simulink model "Automotive_Performance_Package"  (R2022b)
settings: Solver=VariableStepAuto  StartTime=0.0  StopTime=10.0  RelTol=1e-3
libraries: simulink x3, SignalEditorBlockLib x1
settings Model: Creator=Haina Bhawnani  LastModifiedBy=Haina Bhawnani

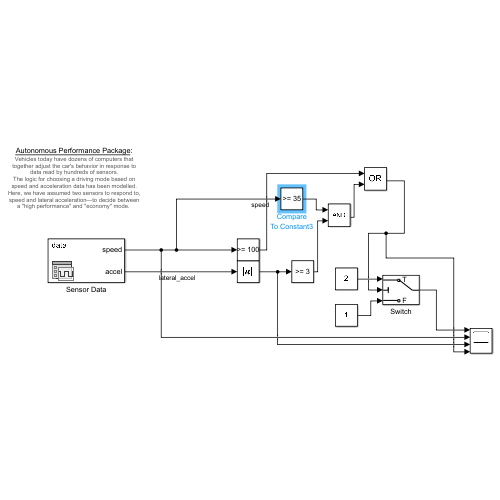
[thumbnail: Simulink's stored preview of the top-level diagram]
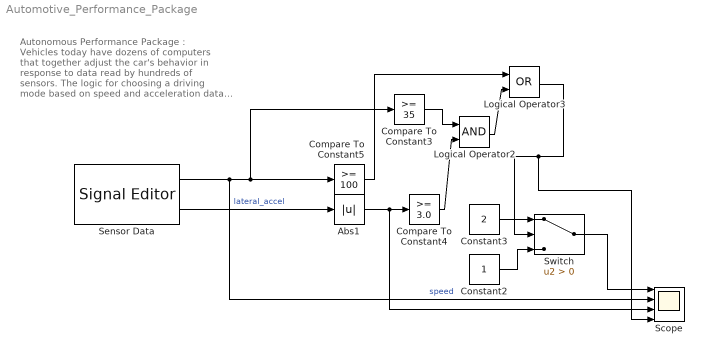
== system Automotive_Performance_Package ==
  note: Autonomous Performance Package :
      | Vehicles today have dozens of computers that together adjust the car's behavior in response to data read by hundreds of sensors.
      | The logic for choosing a driving mode based on speed and acceleration data has been modelled.
      | Here, we have assumed two sensors to respond to, speed and lateral acceleration—to decide between a "high performance" and "economy" mode.
  Abs1 : Abs  SaturateOnIntegerOverflow=off
  Compare To Constant3 : simulink/Logic and Bit Operations/Compare To Constant  relop=>=  const=35  OutDataTypeStr=boolean
  Compare To Constant4 : simulink/Logic and Bit Operations/Compare To Constant  relop=>=  const=3.0  OutDataTypeStr=boolean
  Compare To Constant5 : simulink/Logic and Bit Operations/Compare To Constant  relop=>=  const=100  OutDataTypeStr=boolean
  Constant2 : Constant
  Constant3 : Constant  Value=2
  Logical Operator2 : Logic  AllPortsSameDT=off  OutDataTypeStr=boolean
  Logical Operator3 : Logic  Operator=OR  AllPortsSameDT=off  OutDataTypeStr=boolean
  Scope : Scope  NumInputPorts=4
  Sensor Data : SignalEditorBlockLib/Signal Editor  FileName=signalData.mat  ActiveScenario=data  ActiveSignal=speed  IsBus=off  OutputBusObjectStr=Bus: BusObject  SampleTime=0  Interpolate=off  ZeroCross=off  OutputAfterFinalValue=Setting to zero  Unit=inherit  PreserveSignalName=on
  Switch : Switch  Criteria=u2 > Threshold  SaturateOnIntegerOverflow=off  InputSameDT=off
  wires:
  Compare To Constant5/1 -> Logical Operator3/1
  Logical Operator2/1 -> Logical Operator3/2
  Constant3/1 -> Switch/1
  Compare To Constant3/1 -> Logical Operator2/1
  Sensor Data/2 -> Abs1/1  "lateral_accel"
  Sensor Data/1 -> Scope/2, Compare To Constant3/1, Compare To Constant5/1  "speed"
  Abs1/1 -> Scope/3, Compare To Constant4/1
  Logical Operator3/1 -> Scope/4, Switch/2
  Compare To Constant4/1 -> Logical Operator2/2
  Constant2/1 -> Switch/3
  Switch/1 -> Scope/1
